simulink model "Es3_sim"  (R2024a)
settings: Solver=VariableStepAuto  StartTime=0.0  StopTime=7  RelTol=1e-3
values from neighbouring files (symbols this model uses):
  Alin = J1    [Es3.m]
  Blin = double(subs(jacobian(F,u),[x1,x2,u],[xeq1,ueq]))    [Es3.m]
  Clin1 = double(subs(jacobian(y1,[x1,x2]),[x1,x2,u],[xeq1,ueq]))    [Es3.m]
  Clin2 = double(subs(jacobian(y2,[x1,x2]),[x1,x2,u],[xeq1,ueq]))    [Es3.m]
  ueq = 0    [Es3.m]
  x0 = [3;5]    [Es3.m]
settings Model: Creator=eldemaster  LastModifiedBy=eldemaster
settings RTWCC: GPUComputeCapability=3.5

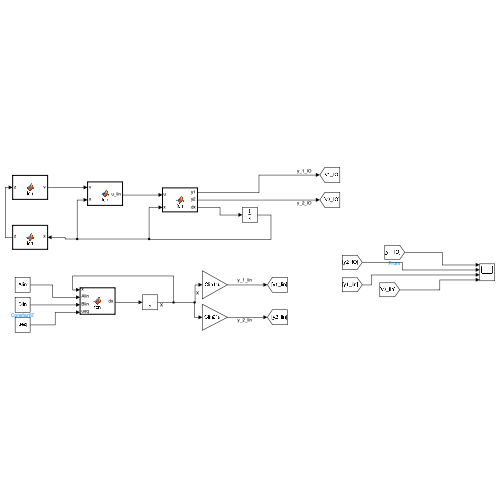
[thumbnail: Simulink's stored preview of the top-level diagram]
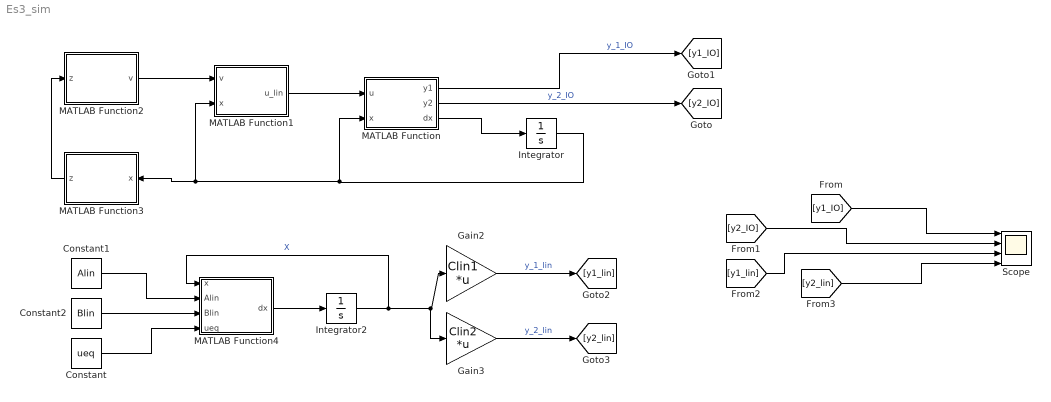
== system Es3_sim ==
  Constant : Constant  Value=ueq
  Constant1 : Constant  Value=Alin
  Constant2 : Constant  Value=Blin
  Gain2 : Gain  Gain=Clin1  Multiplication=Matrix(K*u)
  Gain3 : Gain  Gain=Clin2  Multiplication=Matrix(K*u)
  Integrator : Integrator  InitialCondition=x0
  Integrator2 : Integrator  InitialCondition=[3;5]
  MATLAB Function : MATLAB Function  TreatAsAtomicUnit=on
  MATLAB Function1 : MATLAB Function  TreatAsAtomicUnit=on
  MATLAB Function2 : MATLAB Function  TreatAsAtomicUnit=on
  MATLAB Function3 : MATLAB Function  TreatAsAtomicUnit=on
  MATLAB Function4 : MATLAB Function  TreatAsAtomicUnit=on
  Scope : Scope  NumInputPorts=4
  wires:
  MATLAB Function/3(dx) -> Integrator/1
  Integrator/1 -> MATLAB Function/2(x), MATLAB Function1/2(x), MATLAB Function3/1(x)
  MATLAB Function1/1(u_lin) -> MATLAB Function/1(u)
  MATLAB Function2/1(v) -> MATLAB Function1/1(v)
  MATLAB Function3/1(z) -> MATLAB Function2/1(z)
  MATLAB Function/1(y1) -> [y1_IO]  "y_1_IO"
  MATLAB Function/2(y2) -> [y2_IO]  "y_2_IO"
  Gain2/1 -> [y1_lin]  "y_1_lin"
  Gain3/1 -> [y2_lin]  "y_2_lin"
  Constant/1 -> MATLAB Function4/4(ueq)
  MATLAB Function4/1(dx) -> Integrator2/1
  Integrator2/1 -> Gain3/1, Gain2/1, MATLAB Function4/1(x)  "X"
  Constant1/1 -> MATLAB Function4/2(Alin)
  Constant2/1 -> MATLAB Function4/3(Blin)
  [y1_IO] -> Scope/1
  [y2_IO] -> Scope/2
  [y2_lin] -> Scope/4
  [y1_lin] -> Scope/3

== matlab function Es3_sim/MATLAB Function1 ==
  data: u_lin output; v input; x input
function u_lin  = fcn(v,x)

x1 = x(1);
x2 = x(2);
u_lin =  ((6*x1^2 + 6*x1)*(x1 - 4*x2)- v + 2*x2^2*(6*x1 + 3)*(3*x1^2 + 3*x1))/((6*x1^2 + 6*x1)*(x2 - 3));

== matlab function Es3_sim/MATLAB Function ==
  data: y1 output; y2 output; u input; dx output; x input
function [y1,y2,dx] = fcn(u,x)

x1 = x(1);
x2 = x(2);
dx = [3*(x1^2+x1)*x2; -4*x2+x1-x2*u+3*u];
y1 = 5*x2;
y2 = 2*x1;

== matlab function Es3_sim/MATLAB Function2 ==
  data: v output; z input
function v  = fcn(z)

z1 = z(1);
z2 = z(2);
K = [12.5,7.5];
v = -K(1)*z1-K(2)*z2; % -K*z

== matlab function Es3_sim/MATLAB Function3 ==
  data: z output; x input
function z  = fcn(x)

x1 = x(1);
x2 = x(2);
z = [2*x1; 2*x2*(3*x1^2 + 3*x1)];

== matlab function Es3_sim/MATLAB Function4 ==
  data: x input; Alin input; Blin input; ueq input; dx output
function dx = fcn(x, Alin, Blin, ueq)


dx = Alin*x +Blin*ueq;
